simulink model "sqrttest"  (Simulink 7.7)
settings: Solver=FixedStepDiscrete  StartTime=0.0  StopTime=10.0  FixedStep=1  RelTol=1e-3
settings Model: Creator=hnine  LastModifiedBy=hnine

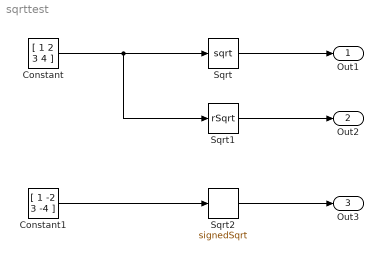
== system sqrttest ==
  Constant : Constant  Value=[ 1 2 3 4 ]
  Constant1 : Constant  Value=[ 1 -2 3 -4 ]
  Sqrt : Sqrt  SaturateOnIntegerOverflow=on
  Sqrt1 : Sqrt  Operator=rSqrt  SaturateOnIntegerOverflow=on
  Sqrt2 : Sqrt  Operator=signedSqrt  SaturateOnIntegerOverflow=on
  Out1 : Outport
  Out2 : Outport  Port=2
  Out3 : Outport  Port=3
  wires:
  Constant/1 -> Sqrt/1, Sqrt1/1
  Sqrt/1 -> Out1/1
  Sqrt1/1 -> Out2/1
  Constant1/1 -> Sqrt2/1
  Sqrt2/1 -> Out3/1
